simulink model "example7"  (Simulink 6.4)
settings: Solver=ode45  StartTime=0.0  StopTime=10  RelTol=1e-3
values from neighbouring files (symbols this model uses):
  Z0 = [0;0;0;0]    [parameter_calRR.m]
undefined symbols (not defined in the file or in its folder): forward_kin_2link, robust_passivity, stateder
settings Model: Creator=rhanz  LastModifiedBy=rhanz  ExtModeAutoUpdateStatusClock=off

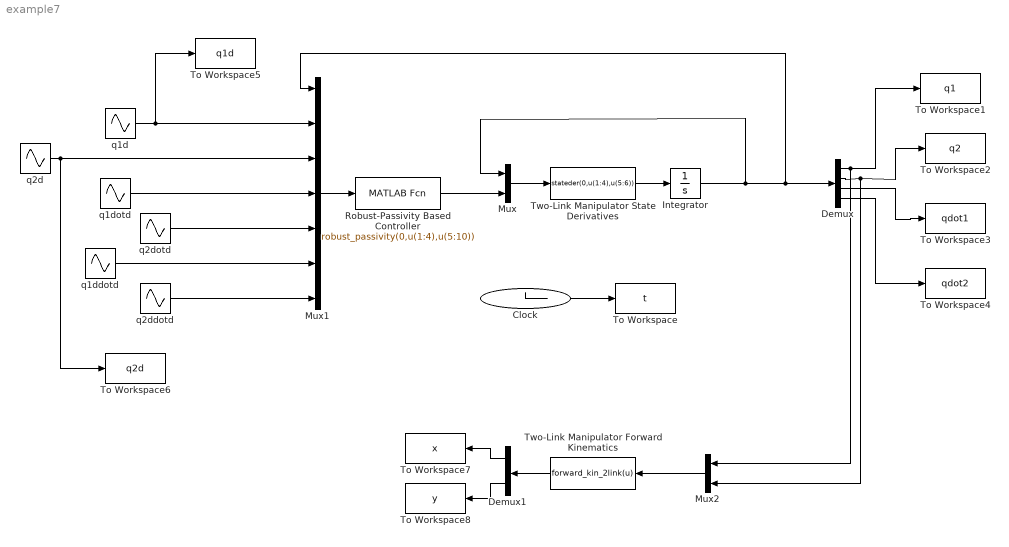
== system example7 ==
  Clock : Clock
      settings: Decimation=10
  Demux : Demux
  Demux1 : Demux  Orientation=left  Outputs=2
  Integrator : Integrator  InitialCondition=Z0
  Mux : Mux  Inputs=2
  Mux1 : Mux  Inputs=7
  Mux2 : Mux  Orientation=left  Inputs=2
  Robust-Passivity Based Controller : MATLABFcn  MATLABFcn=robust_passivity(0,u(1:4),u(5:10))  OutputDimensions=2
  To Workspace : ToWorkspace  VariableName=t  SampleTime=-1  SaveFormat=Array
  To Workspace1 : ToWorkspace  VariableName=q1  SampleTime=-1  SaveFormat=Array
  To Workspace2 : ToWorkspace  VariableName=q2  SampleTime=-1  SaveFormat=Array
  To Workspace3 : ToWorkspace  VariableName=qdot1  SampleTime=-1  SaveFormat=Array
  To Workspace4 : ToWorkspace  VariableName=qdot2  SampleTime=-1  SaveFormat=Array
  To Workspace5 : ToWorkspace  VariableName=q1d  SampleTime=-1  SaveFormat=Array
  To Workspace6 : ToWorkspace  VariableName=q2d  SampleTime=-1  SaveFormat=Array
  To Workspace7 : ToWorkspace  VariableName=x  SampleTime=-1  SaveFormat=Array
  To Workspace8 : ToWorkspace  VariableName=y  SampleTime=-1  SaveFormat=Array
  Two-Link Manipulator Forward Kinematics : MATLABFcn  Orientation=left  MATLABFcn=forward_kin_2link(u)  OutputDimensions=2
  Two-Link Manipulator State Derivatives : MATLABFcn  MATLABFcn=stateder(0,u(1:4),u(5:6))  OutputDimensions=4
  q1d : Sin  SampleTime=0
  q1ddotd : Sin  Phase=pi  SampleTime=0
  q1dotd : Sin  Phase=pi/2  SampleTime=0
  q2d : Sin  Amplitude=0  Phase=pi/2  SampleTime=0
  q2ddotd : Sin  Amplitude=0  Phase=3*pi/2  SampleTime=0
  q2dotd : Sin  Amplitude=0  Phase=pi  SampleTime=0
  wires:
  Two-Link Manipulator State Derivatives/1 -> Integrator/1
  Integrator/1 -> Mux/1, Demux/1, Mux1/1
  Mux/1 -> Two-Link Manipulator State Derivatives/1
  Clock/1 -> To Workspace/1
  Demux/1 -> To Workspace1/1, Mux2/1
  Demux/2 -> To Workspace2/1, Mux2/2
  Demux/3 -> To Workspace3/1
  Demux/4 -> To Workspace4/1
  Robust-Passivity Based Controller/1 -> Mux/2
  Mux1/1 -> Robust-Passivity Based Controller/1
  q1d/1 -> Mux1/2, To Workspace5/1
  q2d/1 -> Mux1/3, To Workspace6/1
  q1dotd/1 -> Mux1/4
  q2dotd/1 -> Mux1/5
  q1ddotd/1 -> Mux1/6
  q2ddotd/1 -> Mux1/7
  Mux2/1 -> Two-Link Manipulator Forward Kinematics/1
  Demux1/1 -> To Workspace7/1
  Demux1/2 -> To Workspace8/1
  Two-Link Manipulator Forward Kinematics/1 -> Demux1/1
